simulink model "ProblemStatement5_Modulation"  (R2020b)
settings: Solver=VariableStepAuto  StartTime=0.0  StopTime=0.01  RelTol=1e-3
settings Model: Creator=amruthashok  LastModifiedBy=nandh

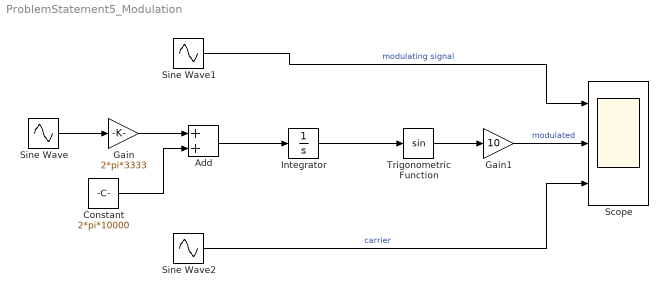
== system ProblemStatement5_Modulation ==
  Add : Sum
  Constant : Constant  Value=2*pi*10000
  Gain : Gain  Gain=2*pi*3333
  Gain1 : Gain  Gain=10
  Integrator : Integrator
  Scope : Scope  NumInputPorts=3
  Sine Wave : Sin  Amplitude=3  Frequency=2*pi*1000  Phase=pi/2  SampleTime=0
  Sine Wave1 : Sin  Amplitude=3  Frequency=2*pi*1000  Phase=pi/2  SampleTime=0
  Sine Wave2 : Sin  Amplitude=10  Frequency=2*pi*10000  SampleTime=0
  Trigonometric Function : Trigonometry
  wires:
  Sine Wave/1 -> Gain/1
  Gain/1 -> Add/1
  Constant/1 -> Add/2
  Add/1 -> Integrator/1
  Integrator/1 -> Trigonometric Function/1
  Gain1/1 -> Scope/2  "modulated"
  Trigonometric Function/1 -> Gain1/1
  Sine Wave1/1 -> Scope/1  "modulating signal"
  Sine Wave2/1 -> Scope/3  "carrier"
